simulink model "MLCSI_2"  (R2024a)
settings: Solver=FixedStepAuto  StartTime=0.0  StopTime=0.3  FixedStep=1e-6  RelTol=1e-3
undefined symbols (not defined in the file): Am, Cf, L, LL, RL
libraries: spsCurrentMeasurementLib x12, spsDiodeLib x12, spsIGBTDiodeLib x12, spsSeriesRLCBranchLib x11, spsVoltageMeasurementLib x8, spsIdealSwitchLib x2, spsControlledCurrentSourceLib x1, spsGroundLib x1, spspowerguiLib x1
(part 2 of 2)

== matlab function MLCSI_2/Lookthrough Table 4_ simplified ==
  settings: updateMethod=DISCRETE  sampleTime=1e-4
  data: va input; S1 output; S2 output; S3 output; S4 output; vb input; vc input; iA input; iB input; iC input; vA_ref input; vB_ref input; vC_ref input; iu1 input; id1 input; Ts input; S5 output; S6 output; S7 output; S8 output; S9 output; S10 output; S11 output; S12 output; ilevel output; F1 output; F2 output; M1 output; M2 output; t output
function [S1,S2,S3,S4,S5,S6,S7,S8,S9,S10,S11,S12,ilevel,F1,F2,M1,M2,t] = fcn(va,vb,vc,iA,iB,iC,vA_ref,vB_ref,vC_ref,iu1,id1,Ts)

tic;
C= 180e-6;
g_opt = inf;
% persistent flag1;
% persistent flag2;
% persistent  module1;
% persistent  module2;
% persistent best_I_level;
% persistent N;


% if isempty(best_I_level)
    best_I_level=1;
% end

% if isempty(module1)
    module1=1;
% end
% 
% if isempty(module2)
    module2=1;
% end
% 
% if isempty(flag1)
    flag1=1;
% end
% 
% if isempty(flag2)
   flag2=1;
% end
% if isempty(N)
%     N=1;
% end



state=[1 0 0 0 1 0;     
       1 0 0 0 0 1;     
       0 1 0 1 0 0;     
       0 1 0 0 0 1;     
       0 0 1 1 0 0;     
       0 0 1 0 1 0;     
       1 0 0 1 0 0;     
       0 1 0 0 1 0;     
       0 0 1 0 0 1];    

inv_current=[   100  -100     0;
               100     0  -100; 
              -100   100     0; 
                 0   100  -100; 
              -100     0   100; 
                 0  -100   100;
               100   -50   -50;
              -100    50    50;
               -50   100   -50;
                50  -100    50;
               -50   -50   100;
                50    50  -100;
                50   -50     0;
               -50    50     0;
                50     0   -50;
               -50     0    50;
                 0    50   -50;
                 0   -50    50;
                ];
   
% if (t==1)
%      if(N==1)

            for i=1:18
                 vA_1 = (Ts/C)*(inv_current(i,1) - iA) + va;
                 vB_1 = (Ts/C)*(inv_current(i,2) - iB) + vb;
                 vC_1 = (Ts/C)*(inv_current(i,3) - iC) + vc;
            
                 g = abs(vA_ref-vA_1)+abs(vB_ref-vB_1)+abs(vC_ref-vC_1);
            
                 if (g<g_opt)
                     g_opt = g;        
                    best_I_level = i;        
                 end
            end            
           
            if (iu1>50)
                if (id1>50)
                    flag1=1;
                end
                if (id1<50)
                    flag1=2;
                end
            end
            if (iu1<50) 
                if (id1>50)
                    flag1=3;
                end
                if (id1<50)
                    flag1=4;
                end 
            end

            if((va>vc)&&(vc>vb))
                flag2=1;
            end
            if((va>vb)&&(vb>vc))
                flag2=2;
            end
            if((vb>va)&&(va>vc))
                flag2=3;
            end
            if((vb>vc)&&(vc>va))
                flag2=4;
            end
            if((vc>vb)&&(vb>va))
                flag2=5;
            end
            if((vc>va)&&(va>vb))
                flag2=6;
            end 

        for br=1:1 
            switch best_I_level
                case 1
                    module1=1;
                    module2=1;
                    break
                case 2
                    module1=2;
                    module2=2;
                    break
                case 3
                    module1=3;
                    module2=3;
                    break
                case 4
                    module1=4;
                    module2=4;
                    break
                case 5
                    module1=5;
                    module2=5;
                    break
                case 6
                    module1=6;
                    module2=6;
                    break

                case 7

                    switch flag1
                    case {1,3}
                        switch flag2
                            case {1,5,6}
                               module1=1;
                               module2=2;
                               break
                            case {2,3,4}
                               module1=2;
                               module2=1;
                               break
                        end

                    case {2,4}
                        switch flag2
                            case {2,3,4}
                               module1=1;
                               module2=2;
                               break
                            case {1,5,6}
                               module1=2;
                               module2=1;
                               break
                        end
                    end

                case 8

                     switch flag1
                    case {1,2}
                        switch flag2
                            case {1,5,6}
                               module1=5;
                               module2=3;
                               break
                            case {2,3,4}
                               module1=3;
                               module2=5;
                               break
                        end

                    case {3,4}
                        switch flag2
                            case {2,3,4}
                               module1=5;
                               module2=3;
                               break
                            case {1,5,6}
                               module1=3;
                               module2=5;
                               break
                        end
                     end

                case 9

                    switch flag1
                    case {1,3}
                        switch flag2
                            case {4,5,6}
                               module1=3;
                               module2=4;
                               break
                            case {1,2,3}
                               module1=4;
                               module2=3;
                               break
                        end

                    case {2,4}
                        switch flag2
                            case {1,2,3}
                               module1=3;
                               module2=4;
                               break
                            case {4,5,6}
                               module1=4;
                               module2=3;
                               break
                        end
                     end   

                case 10

                    switch flag1
                    case {1,2}
                        switch flag2
                            case {4,5,6}
                               module1=6;
                               module2=1;
                               break
                            case {1,2,3}
                               module1=1;
                               module2=6;
                               break
                        end

                    case {3,4}
                        switch flag2
                            case {1,2,3}
                               module1=6;
                               module2=1;
                               break
                            case {4,5,6}
                               module1=1;
                               module2=6;
                               break
                        end
                    end

                case 11

                    switch flag1
                    case {1,3}
                        switch flag2
                            case {3,4,5}
                               module1=5;
                               module2=6;
                               break
                            case {1,2,6}
                               module1=6;
                               module2=5;
                               break
                        end

                    case {2,4}
                        switch flag2
                            case {1,2,6}
                               module1=5;
                               module2=6;
                               break
                            case {3,4,5}
                               module1=6;
                               module2=5;
                               break
                        end
                    end 

                case 12

                    switch flag1
                    case {1,2}
                        switch flag2
                            case {3,4,5}
                               module1=4;
                               module2=2;
                               break
                            case {1,2,6}
                               module1=2;
                               module2=4;
                               break
                        end

                    case {3,4}
                        switch flag2
                            case {1,2,6}
                               module1=4;
                               module2=2;
                               break
                            case {3,4,5}
                               module1=2;
                               module2=4;
                               break
                        end
                    end

                case 13

                    switch flag1
                    case 1 
                        switch flag2
                            case 1                                
                                module1=1;
                                module2=9; 
                                break
                            case 2
                                module1=2;
                                module2=6;
                                break
                            case 3
                                module1=2;
                                module2=6;
                                break
                            case 4                                
                                module1=9;
                                module2=1;
                                break
                            case 5
                                module1=6;
                                module2=2;
                                break
                            case 6
                                module1=6;
                                module2=2;
                                break
                        end
                        
                    case 2
                        switch flag2
                            case 1
                                module1=2;
                                module2=6;
                                break
                            case 2                                
                                module1=1;
                                module2=9;
                                break
                            case 3
                                module1=1;
                                module2=9;
                                break
                            case 4
                                module1=6;
                                module2=2;
                                break
                            case 5
                                module1=9;
                                module2=1;
                                break
                            case 6
                                module1=9;
                                module2=1;
                                break
                        end
                        
                    case 3
                        switch flag2
                            case 1
                                module1=6;
                                module2=2;
                                break
                            case 2                               
                                module1=9;
                                module2=1;
                                break
                            case 3
                                module1=9;
                                module2=1;
                                break
                            case 4
                                module1=2;
                                module2=6;
                                break
                            case 5
                                module1=1;
                                module2=9;
                                break
                            case 6
                                module1=1;
                                module2=9;
                                break
                        end
                                            
                    case 4
                        switch flag2
                            case 1
                                module1=9;
                                module2=1;
                                break
                            case 2
                                module1=6;
                                module2=2;
                                break
                            case 3
                                module1=6;
                                module2=2;
                                break
                            case 4
                                module1=1;
                                module2=9;
                                break
                            case 5
                                module1=2;
                                module2=6;
                                break
                            case 6
                                module1=2;
                                module2=6;
                                break
                        end
                        
                    end

                case 14

                    switch flag1
                    case 1 
                        switch flag2
                            case 1                                
                                module1=9;
                                module2=3;
                                break
                            case 2
                                module1=4;
                                module2=5;
                                break
                            case 3
                                module1=4;
                                module2=5;
                                break
                            case 4                                
                                module1=3;
                                module2=9;
                                break
                            case 5
                                module1=5;
                                module2=4;
                                break
                            case 6
                                module1=5;
                                module2=4;
                                break
                        end
                        
                    case 2
                        switch flag2
                            case 1
                                module1=5;
                                module2=4;
                                break
                            case 2                                
                                module1=3;
                                module2=9;
                                break
                            case 3
                                module1=3;
                                module2=9;
                                break
                            case 4
                                module1=4;
                                module2=5;
                                break
                            case 5
                                module1=9;
                                module2=3;
                                break
                            case 6
                                module1=9;
                                module2=3;
                                break
                        end
                        
                    case 3
                        switch flag2
                            case 1
                                module1=4;
                                module2=5;
                                break
                            case 2                               
                                module1=9;
                                module2=3;
                                break
                            case 3
                                module1=9;
                                module2=3;
                                break
                            case 4
                                module1=5;
                                module2=4;
                                break
                            case 5
                                module1=3;
                                module2=9;
                                break
                            case 6
                                module1=3;
                                module2=9;
                                break
                        end
                                            
                    case 4
                        switch flag2
                            case 1
                                module1=3;
                                module2=9;
                                break
                            case 2
                                module1=5;
                                module2=4;
                                break
                            case 3
                                module1=5;
                                module2=4;
                                break
                            case 4
                                module1=9;
                                module2=3;
                                break
                            case 5
                                module1=4;
                                module2=5;
                                break
                            case 6
                                module1=4;
                                module2=5;
                                break
                        end
                        
                    end

                case 15

                    switch flag1
                    case 1 
                        switch flag2
                            case 1                                
                                module1=1;
                                module2=4;
                                break
                            case 2
                                module1=2;
                                module2=8;
                                break
                            case 3
                                module1=4;
                                module2=1;
                                break
                            case 4                                
                                module1=4;
                                module2=1;
                                break
                            case 5
                                module1=8;
                                module2=2;
                                break
                            case 6
                                module1=1;
                                module2=4;
                                break
                        end
                        
                    case 2
                        switch flag2
                            case 1
                                module1=2;
                                module2=8;
                                break
                            case 2                                
                                module1=1;
                                module2=4; 
                                break
                            case 3
                                module1=8;
                                module2=2;
                                break
                            case 4
                                module1=8;
                                module2=2;
                                break
                            case 5
                                module1=4;
                                module2=1;
                                break
                            case 6
                                module1=2;
                                module2=8; 
                                break
                        end
                        
                    case 3
                        switch flag2
                            case 1
                                module1=8;
                                module2=2;
                                break
                            case 2                               
                                module1=4;
                                module2=1;
                                break
                            case 3
                                module1=2;
                                module2=8;
                                break
                            case 4
                                module1=2;
                                module2=8;
                                break
                            case 5
                                module1=1;
                                module2=4;
                                break
                            case 6
                                module1=8;
                                module2=2;
                                break
                        end
                                            
                    case 4
                        switch flag2
                            case 1
                                module1=4;
                                module2=1;
                                break
                            case 2
                                module1=8;
                                module2=2;
                                break
                            case 3
                                module1=1;
                                module2=4;
                                break
                            case 4
                                module1=1;
                                module2=4;
                                break
                            case 5
                                module1=2;
                                module2=8;
                                break
                            case 6
                                module1=4;
                                module2=1;
                                break
                        end
                        
                    end

                case 16

                    switch flag1
                    case 1 
                        switch flag2
                            case 1                                
                                module1=6;
                                module2=3;
                                break
                            case 2
                                module1=8;
                                module2=5;
                                break
                            case 3
                                module1=3;
                                module2=6;
                                break
                            case 4                                
                                module1=3;
                                module2=6;
                                break
                            case 5
                                module1=5;
                                module2=8;
                                break
                            case 6
                                module1=6;
                                module2=3;
                                break
                        end
                        
                    case 2
                        switch flag2
                            case 1
                                module1=5;
                                module2=8;
                                break
                            case 2                                
                                module1=3;
                                module2=6;
                                break
                            case 3
                                module1=8;
                                module2=5;
                                break
                            case 4
                                module1=8;
                                module2=5;
                                break
                            case 5
                                module1=6;
                                module2=3;
                                break
                            case 6
                                module1=5;
                                module2=8;
                                break
                        end
                        
                    case 3
                        switch flag2
                            case 1
                                module1=8;
                                module2=5;
                                break
                            case 2                               
                                module1=6;
                                module2=3;
                                break
                            case 3
                                module1=5;
                                module2=8;
                                break
                            case 4
                                module1=5;
                                module2=8;
                                break
                            case 5
                                module1=3;
                                module2=6;
                                break
                            case 6
                                module1=8;
                                module2=5;
                                break
                        end
                                            
                    case 4
                        switch flag2
                            case 1
                                module1=3;
                                module2=6;
                                break
                            case 2
                                module1=5;
                                module2=8;
                                break
                            case 3
                                module1=6;
                                module2=3;
                                break
                            case 4
                                module1=6;
                                module2=3;
                                break
                            case 5
                                module1=8;
                                module2=5;
                                break
                            case 6
                                module1=3;
                                module2=6;
                                break
                        end
                        
                    end

                case 17

                    switch flag1
                    case 1 
                        switch flag2
                            case 1                                
                                module1=2;
                                module2=3;
                                break
                            case 2
                                module1=2;
                                module2=3;
                                break
                            case 3
                                module1=4;
                                module2=7;
                                break
                            case 4                                
                                module1=3;
                                module2=2;
                                break
                            case 5
                                module1=3;
                                module2=2;
                                break
                            case 6
                                module1=7;
                                module2=4;
                                break
                        end
                        
                    case 2
                        switch flag2
                            case 1
                                module1=7;
                                module2=4;
                                break
                            case 2                                
                                module1=7;
                                module2=4;
                                break
                            case 3
                                module1=3;
                                module2=2;
                                break
                            case 4
                                module1=4;
                                module2=7;
                                break
                            case 5
                                module1=4;
                                module2=7;
                                break
                            case 6
                                module1=2;
                                module2=3;
                                break
                        end
                        
                    case 3
                        switch flag2
                            case 1
                                module1=4;
                                module2=7;
                                break
                            case 2                               
                                module1=4;
                                module2=7;
                                break
                            case 3
                                module1=2;
                                module2=3;
                                break
                            case 4
                                module1=7;
                                module2=4;
                                break
                            case 5
                                module1=7;
                                module2=4;
                                break
                            case 6
                                module1=3;
                                module2=2;
                                break
                        end
                                            
                    case 4
                        switch flag2
                            case 1
                                module1=3;
                                module2=2;
                                break
                            case 2
                                module1=3;
                                module2=2;
                                break
                            case 3
                                module1=7;
                                module2=4;
                                break
                            case 4
                                module1=2;
                                module2=3;
                                break
                            case 5
                                module1=2;
                                module2=3;
                                break
                            case 6
                                module1=4;
                                module2=7;
                                break
                        end
                        
                    end

                case 18

                    switch flag1
                    case 1 
                        switch flag2
                            case 1                                
                                module1=1;
                                module2=5;
                                break
                            case 2
                                module1=1;
                                module2=5;
                                break
                            case 3
                                module1=7;
                                module2=6;
                                break
                            case 4                                
                                module1=5;
                                module2=1;
                                break
                            case 5
                                module1=5;
                                module2=1;
                                break
                            case 6
                                module1=6;
                                module2=7;
                                break
                        end
                        
                    case 2
                        switch flag2
                            case 1
                                module1=7;
                                module2=6;
                                break
                            case 2                                
                                module1=7;
                                module2=6;
                                break
                            case 3
                                module1=1;
                                module2=5;
                                break
                            case 4
                                module1=6;
                                module2=7;
                                break
                            case 5
                                module1=6;
                                module2=7;
                                break
                            case 6
                                module1=5;
                                module2=1;
                                break
                        end
                        
                    case 3
                        switch flag2
                            case 1
                                module1=6;
                                module2=7;
                                break
                            case 2                               
                                module1=6;
                                module2=7;
                                break
                            case 3
                                module1=5;
                                module2=1;
                                break
                            case 4
                                module1=7;
                                module2=6;
                                break
                            case 5
                                module1=7;
                                module2=6;
                                break
                            case 6
                                module1=1;
                                module2=5;
                                break
                        end
                                            
                    case 4
                        switch flag2
                            case 1
                                module1=5;
                                module2=1;
                                break
                            case 2
                                module1=5;
                                module2=1;
                                break
                            case 3
                                module1=6;
                                module2=7;
                                break
                            case 4
                                module1=1;
                                module2=5;
                                break
                            case 5
                                module1=1;
                                module2=5;
                                break
                            case 6
                                module1=7;
                                module2=6;
                                break
                        end
                        
                    end

            end

        end

%    N=0;
%      else
%      end
%  else
%      N=1;
%  end

       

    S1 = state(module1,1);
    S2 = state(module1,2);
    S3 = state(module1,3);
    S4 = state(module1,4);
    S5 = state(module1,5);
    S6 = state(module1,6);

    S7 = state(module2,1);
    S8 = state(module2,2);
    S9 = state(module2,3);
    S10 = state(module2,4);
    S11 = state(module2,5);
    S12 = state(module2,6);
    t=toc;
    ilevel=best_I_level;
    F1=flag1;
    F2=flag2;
    M1=module1;
    M2=module2;

== matlab function MLCSI_2/Formula Calculation1 ==
  settings: updateMethod=DISCRETE  sampleTime=1e-4
  data: vA input; S1 output; S2 output; S3 output; S4 output; vB input; vC input; iA input; iB input; iC input; vA_ref input; vB_ref input; vC_ref input; iu1 input; iu2 input; id1 input; id2 input; Ts input; S5 output; S6 output; S7 output; S8 output; S9 output; S10 output; S11 output; S12 output; t output
function [S1,S2,S3,S4,S5,S6,S7,S8,S9,S10,S11,S12,t] = fcn(vA,vB,vC,iA,iB,iC,vA_ref,vB_ref,vC_ref,iu1,iu2,id1,id2,Ts)

tic;
L= 30e-3;
C= 180e-6;
lambda1=0.925;
lambda2=0.025;

state=[1 0 0 0 1 0;     
       1 0 0 0 0 1;     
       0 1 0 1 0 0;     
       0 1 0 0 0 1;    
       0 0 1 1 0 0;     
       0 0 1 0 1 0;    
       1 0 0 1 0 0;     
       0 1 0 0 1 0;    
       0 0 1 0 0 1];   

  
% persistent x_opt1;
% persistent x_opt2;
% persistent N;


% if isempty(x_opt1)
     x_opt1=0;
% end

% if isempty(x_opt2)
     x_opt2=0;
% end

% if isempty(N)
%     N=1;
% end

g_opt = inf;

% if (t==1)
%      if(N==1)

        for i=1:9
            for j= 1:9
                
                i_inva = state(i,1)*iu1+state(j,1)*iu2-(state(i,4)*id1+state(j,4)*id2);
                i_invb = state(i,2)*iu1+state(j,2)*iu2-(state(i,5)*id1+state(j,5)*id2);
                i_invc = state(i,3)*iu1+state(j,3)*iu2-(state(i,6)*id1+state(j,6)*id2);

                vun1 = state(i,1)*vA + state(i,2)*vB + state(i,3)*vC;
                vun2 = state(j,1)*vA + state(j,2)*vB + state(j,3)*vC;

                vnd1 = -(state(i,4)*vA + state(i,5)*vB + state(i,6)*vC);
                vnd2 = -(state(j,4)*vA + state(j,5)*vB + state(j,6)*vC);

                iu1_1 = (Ts/(2*L))*(vun2-vun1) + iu1;
                iu2_1 = (Ts/(2*L))*(vun1-vun2) + iu2;
                id1_1 = (Ts/(2*L))*(vnd2-vnd1) + id1;
                id2_1 = (Ts/(2*L))*(vnd1-vnd2) + id2;


                 vA_1 = (Ts/C)*(i_inva - iA) + vA;
                 vB_1 = (Ts/C)*(i_invb - iB) + vB;
                 vC_1 = (Ts/C)*(i_invc - iC) + vC;
                
                g = lambda1*(abs(vA_ref-vA_1)+abs(vB_ref-vB_1)+abs(vC_ref-vC_1))/900+...
                    lambda2*(abs(iu1_1-50)+abs(iu2_1-50)+abs(id1_1-50)+abs(id2_1-50))/50;
                    
            
                    if (g<g_opt)
                        g_opt = g;
                        x_opt1 = i;
                        x_opt2 = j;
                    end
                
            end
        end

%          N=0;
%      else
%      end
%  else
%      N=1;
%  end


    S1 = state(x_opt1,1);
    S2 = state(x_opt1,2);
    S3 = state(x_opt1,3);
    S4 = state(x_opt1,4);
    S5 = state(x_opt1,5);
    S6 = state(x_opt1,6);

    S7 = state(x_opt2,1);
    S8 = state(x_opt2,2);
    S9 = state(x_opt2,3);
    S10 = state(x_opt2,4);
    S11 = state(x_opt2,5);
    S12 = state(x_opt2,6);

    % module1=x_opt1;
    % module2=x_opt2;

    t=toc;
